simulink model "DOF2"  (R2021a)
settings: Solver=VariableStepAuto  StartTime=0.0  StopTime=15  RelTol=1e-3
settings Model: Creator=monal  LastModifiedBy=monal

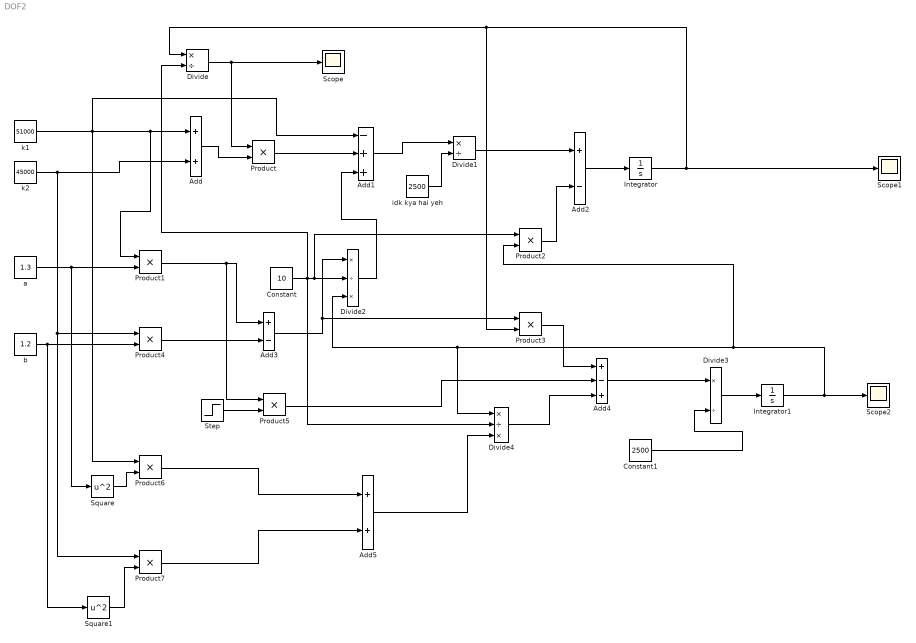
== system DOF2 ==
  Add : Sum
  Add1 : Sum  Inputs=-++
  Add2 : Sum  Inputs=+-
  Add3 : Sum  Inputs=+-
  Add4 : Sum  Inputs=+-+
  Add5 : Sum
  Constant : Constant  Value=10
  Constant1 : Constant  Value=2500
  Divide : Product  Inputs=*/
  Divide1 : Product  Inputs=*/
  Divide2 : Product  Inputs=*/*
  Divide3 : Product  Inputs=*/
  Divide4 : Product  Inputs=*/*
  Integrator : Integrator
  Integrator1 : Integrator
  Product{,1..7} (8 alike) : Product
  Scope : Scope
  Scope1 : Scope
  Scope2 : Scope
  Square : Math  Operator=square  SaturateOnIntegerOverflow=on
  Square1 : Math  Operator=square  SaturateOnIntegerOverflow=on
  Step : Step  Time=0  After=0.4  SampleTime=0
  a : Constant  Value=1.3
  b : Constant  Value=1.2
  idk kya hai yeh : Constant  Value=2500
  k1 : Constant  Value=51000
  k2 : Constant  Value=45000
  wires:
  k1/1 -> Product6/1, Add1/1, Product1/1, Add/1
  k2/1 -> Product4/1, Product7/1, Add/2
  Add/1 -> Product/2
  Divide/1 -> Product/1, Scope/1
  Product/1 -> Add1/2
  Add1/1 -> Divide1/1
  idk kya hai yeh/1 -> Divide1/2
  Divide1/1 -> Add2/1
  Add2/1 -> Integrator/1
  Integrator/1 -> Divide/1, Product3/2, Scope1/1
  a/1 -> Square/1, Product1/2
  Divide2/1 -> Add1/3
  Product2/1 -> Add2/2
  Constant/1 -> Divide4/2, Product2/1, Divide2/2, Divide/2
  b/1 -> Square1/1, Product4/2
  Product4/1 -> Add3/2
  Product1/1 -> Product5/1, Add3/1
  Add3/1 -> Product3/1, Divide2/1
  Product3/1 -> Add4/1
  Add4/1 -> Divide3/1
  Product5/1 -> Add4/2
  Step/1 -> Product5/2
  Divide3/1 -> Integrator1/1
  Integrator1/1 -> Product2/2, Divide4/1, Divide2/3, Scope2/1
  Constant1/1 -> Divide3/2
  Divide4/1 -> Add4/3
  Add5/1 -> Divide4/3
  Product6/1 -> Add5/1
  Product7/1 -> Add5/2
  Square/1 -> Product6/2
  Square1/1 -> Product7/2
